simulink model "Line_Test"  (R2025b)
settings: Solver=FixedStepAuto  StartTime=0.0  StopTime=inf  RelTol=1e-3
settings Model: SimulationMode=external  Creator=kueh_js  LastModifiedBy=kueh_js
settings OptimizationCC: OptimizeBlockIOStorage=off  EnhancedBackFolding=on  PassReuseOutputArgsThreshold=0.0  ZeroExternalMemoryAtStartup=off  ZeroInternalMemoryAtStartup=off  OptimizeBlockOrder=speed  DifferentSizesBufferReuse=on
settings DebuggingCC: ParameterTunabilityLossMsg=error
settings HardwareCC: ProdBitPerLong=64.0  ProdHWDeviceType=Intel->x86-64 (Linux 64)
settings SFSimCC: MATLABDynamicMemAlloc=off  SimTargetLang=C++  SimDLTargetLibrary=mkl-dnn
settings RTWCC: GenCodeOnly=on  Toolchain=GNU gcc/g++ | gmake (64-bit Linux)  TargetLang=C++
settings CodeAppCC: ForceParamTrailComments=on  OperatorAnnotations=on  MATLABSourceComments=on
settings GRTTargetCC: TargetLangStandard=C++20 (ISO)  MatFileLogging=off  CodeInterfacePackaging=C++ class

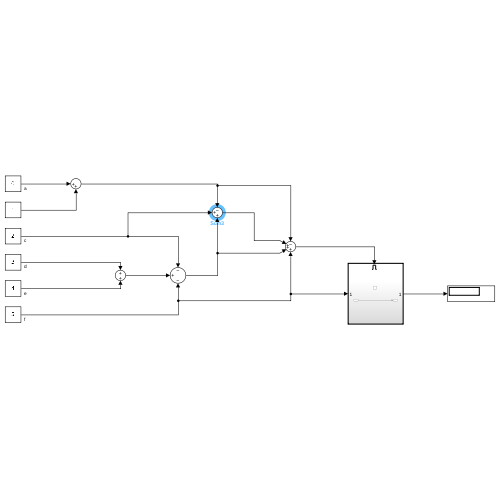
[thumbnail: Simulink's stored preview of the top-level diagram]
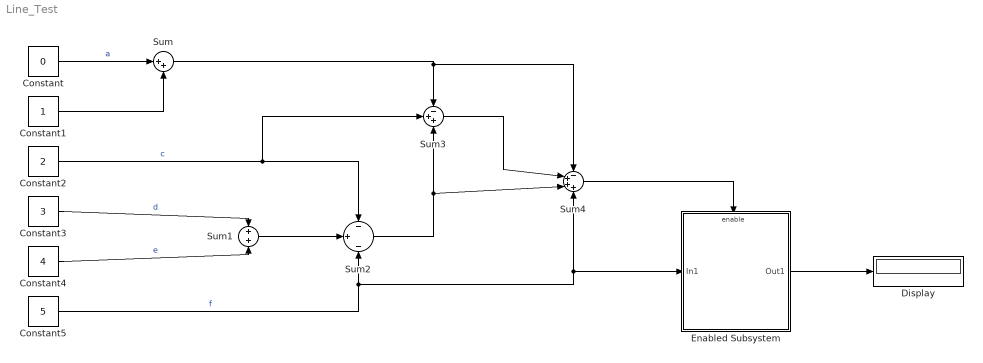
== system Line_Test ==
  Constant : Constant  Value=0
  Constant1 : Constant
  Constant2 : Constant  Value=2
  Constant3 : Constant  Value=3
  Constant4 : Constant  Value=4
  Constant5 : Constant  Value=5
  Display : Display
  Enabled Subsystem : Subsystem  TreatAsAtomicUnit=on
  Sum : Sum  Inputs=|++
  Sum1 : Sum
  Sum2 : Sum  Inputs=-|+|-
  Sum3 : Sum  Inputs=-++
  Sum4 : Sum  Inputs=-+++
  wires:
  Constant/1 -> Sum/1  "a"
  Constant1/1 -> Sum/2
  Constant3/1 -> Sum1/1  "d"
  Constant4/1 -> Sum1/2  "e"
  Constant2/1 -> Sum3/2, Sum2/1  "c"
  Sum1/1 -> Sum2/2
  Constant5/1 -> Sum4/4, Enabled Subsystem/1(In1), Sum2/3  "f"
  Sum2/1 -> Sum4/3, Sum3/3
  Sum/1 -> Sum4/1, Sum3/1
  Sum3/1 -> Sum4/2
  Sum4/1 -> Enabled Subsystem/Enable
  Enabled Subsystem/1(Out1) -> Display/1

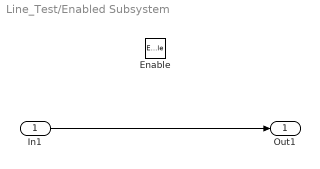
== system Line_Test/Enabled Subsystem ==
  In1 : Inport
  Enable : EnablePort
  Out1 : Outport
  wires:
  In1/1 -> Out1/1
